simulink model "chernovik"  (R2018a)
settings: Solver=VariableStepAuto  StartTime=0.0  StopTime=10.0  RelTol=1e-3
settings Model: Creator=user  LastModifiedBy=user

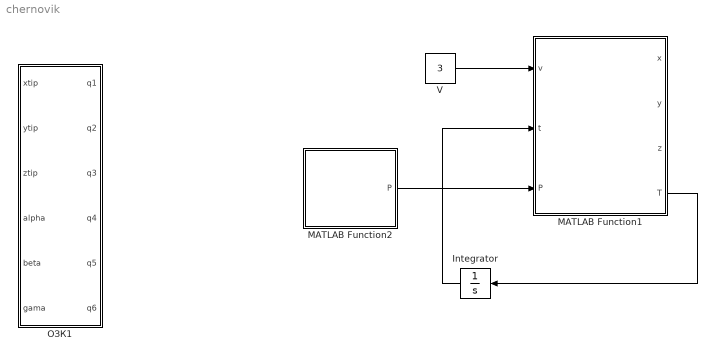
== system chernovik ==
  Integrator : Integrator
  MATLAB Function1 : MATLAB Function  TreatAsAtomicUnit=on
  MATLAB Function2 : MATLAB Function  TreatAsAtomicUnit=on
  V : Constant  Value=3
  ОЗК1 : MATLAB Function  TreatAsAtomicUnit=on
  wires:
  V/1 -> MATLAB Function1/1(v)
  MATLAB Function2/1(P) -> MATLAB Function1/3(P)
  MATLAB Function1/4(T) -> Integrator/1
  Integrator/1 -> MATLAB Function1/2(t)

== matlab function chernovik/MATLAB Function2 ==
  data: P output
function P = fcn()
%  Px   = [10 12.5 15 15 15 12.5 10 7.5 5 5 5 7.5 10 12.5 15 15 15 12.5 10 7.5 5 5 5 7.5];
%  Py   = [5 5 7.5 10 12.5 15 15 15 12.5 10 7.5 5 5 5 7.5 10 12.5 15 15 15 12.5 10 7.5 5]; 
%  Pz   = [6 6 6 6 6 6 6 6 6 6 6 6 6 6 6 6 6 6 6 6 6 6 6 6];
t=0;
i=1;
Px=zeros(1,63);
Py=Px;
Pz=Py;
while t<2*pi
x=0.2*cos(t)+0.8;
y=0.2*sin(t);
z=0.4;

Px(i)=x;
Py(i)=y;
Pz(i)=z;

t=t+0.1;
i=i+1;
end
P=[Px;Py;Pz];
end

== matlab function chernovik/MATLAB Function1 ==
  data: x output; v input; y output; t input; P input; z output; T output
function [x,y,z,T] = TargetPosition(v,t,P)

  i=2;
  for k = 1:1:length(P)-4
    if (t>k)
     i = k+2;
    end
  end
  t = t - i+2;

    Ak=zeros(1,3);
    Bk=zeros(1,3);
    Ck=zeros(1,3);
    Dk=zeros(1,3);
    F=zeros(1,3);
    S=zeros(1,3);
    
    for j=1:3
    Ak(j)=(-P(j,i-1)+3*P(j,i)-3*P(j,i+1)+P(j,i+2))/6;
    Bk(j)=(3*P(j,i-1)-6*P(j,i)+3*P(j,i+1))/6;
    Ck(j)=(-3*P(j,i-1)+3*P(j,i+1))/6;
    Dk(j)=(P(j,i-1)+4*P(j,i)+P(j,i+1))/6;
    F(j)=3*Ak(j)*t^2+2*Bk(j)*t+Ck(j);
    S(j)=Ak(j)*t^3+Bk(j)*t^2+Ck(j)*t+Dk(j);
    end
    T=v/sqrt(F(1)^2+F(2)^2+F(3)^2);
    
    x=S(1);
    y=S(2);
    z=S(3);



end

== matlab function chernovik/ОЗК1 ==
  data: xtip input; q1 output; ytip input; ztip input; alpha input; beta input; gama input; q2 output; q3 output; q4 output; q5 output; q6 output
function [q1,q2,q3,q4,q5,q6] = INVERSE(xtip,ytip,ztip,alpha,beta,gama) 

% DECLERATION OF THE ROBOT PARAMETER
d1 = 0.352;
a1 = 0.070;
a2 = 0.360;
d4 = 0.380;
d6=0.065;


NOSOLUTION=1000;

% THIS PROGRAM IS DESIGNED TO SOLVE THE INVERSE WITH RESPECT TO Porg6 OR TCP ACCORDING TO USER SELECTION
% sel = input ('TO SOLVE THE INVERSE WITH RESPECT TO FRAME6 PRESS 1 WHILE, TO SOLVE THE INVERSE WITH RESPECT TO TCP ENTER 2: ');
% if (sel == 1)
% d6 = 0;
% elseif (sel == 2)
% d6 = 65;
% else
% d6= 65;
% end

% USER INTERFACE
% xtip = input ('PLEASE ENTER THE GOAL POSTION X = ');
% ytip = input ('PLEASE ENTER THE GOAL POSTION y = ');
% ztip = input ('PLEASE ENTER THE GOAL POSTION z = ');
% alpha= input ('PLEASE ENTER THE VALUE OF alpha IN DEGREE = ');
% beta = input ('PLEASE ENTER THE VALUE OF beta IN DEGREE = ');
% gama = input ('PLEASE ENTER THE VALUE OF gama IN DEGREE = ');


% CALCULATING ALL THE POSSIBLE VALUES FOR THETA1
theta1= atan2 (ytip,xtip);
theta11= pi + theta1;
THETA1 = theta1 * 180/pi;
THETA11= theta11 * 180/pi;

% CALCULATING ALL THE POSSIBLE VALUES FOR THETA3
s = (ztip - d1);
r = sqrt((xtip - a1*cos (theta1))^2 +(ytip - a1*sin(theta1))^2);
czeta = (r^2 + s^2 - (a2)^2 - (d4 + d6)^2)/(2 * a2 *(d4 + d6));

% SINGULARTIY CONDTION, CHECK IF THE POSTION WITHIN THE WORKSPACE OR NOT
if (abs(czeta) <= 1)
szeta = sqrt(1-(czeta)^2);
szeta1 = -szeta;
zeta= atan2(szeta,czeta);
zeta1= atan2(szeta1,czeta);
theta3 = -(pi/2 + zeta);
theta33 = -(pi/2 + zeta1);
THETA3 = conversion( theta3,50,-230);
THETA33 = conversion( theta33,50,-230);
else
theta3 = NOSOLUTION; 


theta33= NOSOLUTION;
THETA3 = (NOSOLUTION);
THETA33 = (NOSOLUTION);
end
s = (ztip - d1);
r = sqrt((xtip - a1*cos (theta11))^2 +(ytip - a1*sin(theta11))^2);
czetai = (r^2 + s^2 - (a2)^2 - (d4 + d6)^2)/(2 * a2 *(d4 + d6));

% SINGULARTIY CONDTION, CHECK IF THE POSTION WITHIN THE WORKSPACE OR NOT
if (abs(czetai) <= 1)
szetai = sqrt(1-(czetai)^2);
szeta1i = -szetai;
zetai= atan2(szetai,czetai);
zeta1i= atan2(szeta1i,czetai);
theta3i = -(pi/2 + zetai);
theta33i = -(pi/2 + zeta1i);
THETA3i = conversion( theta3i,50,-230);
THETA33i = conversion( theta33i,50,-230);
else
theta3i=NOSOLUTION;
theta33i=NOSOLUTION;
THETA3i = (NOSOLUTION);
THETA33i = (NOSOLUTION);
end
% CALCULATING ALL THE POSSIBLE VALUES FOR THETA2
if (theta3 == NOSOLUTION)
THETA2 = (NOSOLUTION);
THETA22 = (NOSOLUTION);
else
theta2 = THE2(xtip,ytip,ztip,theta1,zeta);
theta22 = THE2COMP(xtip,ytip,ztip,theta1,zeta);
THETA2 = conversion( theta2,110,-90);
THETA22 = conversion( theta22,110,-90);
end
if (theta33 == NOSOLUTION)
THETA2i = (NOSOLUTION);
THETA22i = (NOSOLUTION);
else
theta2i = THE2(xtip,ytip,ztip,theta1,zeta1);
theta22i = THE2COMP(xtip,ytip,ztip,theta1,zeta1);
THETA2i = conversion( theta2i,110,-90);
THETA22i = conversion( theta22i,110,-90);
end
if (theta3i == NOSOLUTION)
THETA2j = (NOSOLUTION);
THETA22j = (NOSOLUTION);
else
theta2j = THE2(xtip,ytip,ztip,theta11,zetai); 

theta22j = THE2COMP(xtip,ytip,ztip,theta11,zetai);
THETA2j = conversion( theta2j,100,-90);
THETA22j = conversion( theta22j,100,-90);
end
if (theta33i == NOSOLUTION)
THETA2k = (1000);
THETA22k = (1000);
else
theta2k = THE2(xtip,ytip,ztip,theta11,zeta1i);
theta22k = THE2COMP(xtip,ytip,ztip,theta11,zeta1i);
THETA2k = conversion( theta2k,110,-90);
THETA22k = conversion( theta22k,110,-90);
end
% DISPLAY ALL THE POSSIBLE EIGHT SOLUTIONS, NOTE THAT EVERY TWO SOLUTIONS FORM ONLY ONE SOLUTION SET
% disp ( ' THETA 1,2,3 SOLUTIONS')
% disp ( ' SET 1')

SOL1 =[ THETA1, THETA2, THETA3];
SOL2 =[ THETA1, THETA22, THETA3];
% disp ( ' SET 2')
SOL3 =[ THETA1, THETA2i, THETA33];
SOL4 =[ THETA1, THETA22i, THETA33];
% disp ( ' SET 3')
SOL5 =[ THETA11, THETA2j, THETA3i];
SOL6 =[ THETA11, THETA22j, THETA3i];
% disp ( ' SET 4')
SOL7 =[ THETA11, THETA2k, THETA33i];
SOL8 =[ THETA11, THETA22k, THETA33i];

% SOLVING THE SECOND KINEMATIC SUB-PROBLEM (ORIENTATION)
alpha = alpha * pi/180;
beta = beta * pi/180;
gama = gama * pi/180;
R60 = [cos(alpha).*cos(beta), (cos(alpha).*sin(beta).*sin(gama))- sin(alpha).*cos(gama),(cos(alpha).*sin(beta).*cos(gama)) + sin(alpha).*sin(gama) ;
 sin(alpha).*cos(beta), (sin(alpha).*sin(beta).*sin(gama)) + cos(alpha).*cos(gama),(sin(alpha).*sin(beta).*cos(gama)) - cos(alpha).*sin(gama) ;
 - sin(beta), cos(beta).*sin(gama), cos(beta).*sin(gama)];
R30 = [cos(theta1).*cos(theta2+theta3), -cos(theta1).*sin(theta2+theta3), sin(theta1);
 sin(theta1).*cos(theta2+theta3), -sin(theta1).*sin(theta2+theta3), cos(theta1);
 -sin(theta2+theta3), -cos(theta2+theta3), 0 ] ;
 

RT30= transpose (R30);
R63 = RT30 * R60 ;
g11 = R63 (1,1);
g12 = R63 (1,2);
g23 = R63 (2,3);
g31 = R63 (3,1);
g32 = R63 (3,2);
g33 = R63 (3,3);

% THETA 4,5,6 CALCULATION
theta5 = atan2 ( sqrt((g31)^2 +(g32)^2), g33);
if(theta5 == 0)
THETA4= 0;
THETA5= 0;
theta6 = atan2 (-g12, g11);
THETA6= theta6*180/pi;
elseif (theta5 == pi)
THETA4= 0;
THETA5= 0;
theta6 = atan2 (g12,-g11);
THETA6= theta6*180/pi;
else
theta4 = atan2 (g32/ sin (theta5), - g31/ sin (theta5));
theta6 = atan2 (g23/ sin (theta5), g31/ sin (theta5));
THETA4= conversion( theta4,200,-200);
THETA5= conversion( theta5,115,-115);
THETA6= conversion( theta6,400,-400);

% FLIPPED POSTION
theta44 = theta4 + pi;
theta55 = -theta5;
theta66 = theta6+pi;
THETA44= conversion( theta44,200,-200);
THETA55= conversion( theta55,115,-115);
THETA66= conversion( theta66,400,-400);
% disp ( ' THETA 4,5,6 SOLUTIONS')
Solution1 = [THETA4,THETA5,THETA6];
Solution2 = [THETA44,THETA55,THETA66];
end

SOL1=SOL1/180*pi;
Solution1=Solution1/180*pi;
% if theta1~=NOSOLUTION&&theta2~=NOSOLUTION&&theta3~=NOSOLUTION
 q1=SOL1(1);
 q2=SOL1(2);
 q3=SOL1(3);
q4=Solution1(1);
q5=Solution1(2);
q6=Solution1(3);


function RES = THE2(xtip,ytip,ztip,theta1,zeta)
 s = (ztip - d1);
 r = sqrt((xtip - a1*cos (theta1))^2 +(ytip - a1*sin(theta1))^2);
omega = atan2 (s, r);
lenda = atan2 (( d4+d6) * sin (zeta) , a2+( d4+d6)* cos (zeta));
RES = - ((omega - lenda)- ( pi/2)) ;
end

% SECOND POSSIBLE SOLUTION OF THETA2 FUNCTION
function RES1 = THE2COMP(xtip,ytip,ztip,theta1,zeta)
s = (ztip - d1);
r = - sqrt((xtip - a1*cos (theta1))^2 +(ytip - a1*sin(theta1))^2);
omega = atan2 (s, r);
lenda = atan2 (( d4+d6) * sin (zeta) , a2+( d4+d6)* cos (zeta));
RES1 = - ((omega - lenda) - ( pi/2));
end
% JOINT ANGLES LIMIT FUNCTION
function OUT = conversion( theta,upperlimit,lowerlimit)
upperlimit = upperlimit * pi / 180;
lowerlimit = lowerlimit * pi / 180;
if (theta > upperlimit)
OUT = (NOSOLUTION);
elseif (theta < lowerlimit)
OUT = (NOSOLUTION);
else
OUT = theta * 180 / pi;
end
end
end
